simulink model "ScriptDemo"  (R2022b)
settings: configuration reference "TmVcThermal_Configuration_sub" (kept outside this file)
undefined symbols (not defined in the file): aaaa, bbbb, cTmComprCtrl_D_u8HvacFlowTable_db, cTmComprCtrl_D_u8HvacFlowTable_sw, cTmComprCtrl_n_i16ChillCmpIMax, cTmComprCtrl_n_i16ChillCmpIMin, cTmComprCtrl_n_i16ChillCmpIMin666, cTmComprCtrl_n_i16ChillCmpPMax, cTmComprCtrl_n_i16ChillCmpPMin, cTmComprCtrl_n_i16CmpChillCoolRpmKiMax, cTmComprCtrl_n_i16CmpChillCoolRpmKiMin, cTmComprCtrl_n_i16CmpChillCoolRpmKpMax, cTmComprCtrl_n_i16CmpChillCoolRpmKpMin, cTmComprCtrl_n_i16CmpCoolRpmKiMax, cTmComprCtrl_n_i16CmpCoolRpmKiMin, cTmComprCtrl_n_i16CmpCoolRpmKpMax, cTmComprCtrl_n_i16CmpCoolRpmKpMin, cTmComprCtrl_n_i16SM4CmpHeatKiMax, cTmComprCtrl_n_i16SM4CmpHeatKiMin, cTmComprCtrl_n_i16SM4CmpHeatKpMax, cTmComprCtrl_n_i16SM4CmpHeatKpMin, cTmComprCtrl_n_i16SM5CmpHeatKiMax, cTmComprCtrl_n_i16SM5CmpHeatKiMin, cTmComprCtrl_n_i16SM5CmpHeatKpMax, cTmComprCtrl_n_i16SM5CmpHeatKpMin, cTmComprCtrl_n_i16SM6CmpHeatKiMax, cTmComprCtrl_n_i16SM6CmpHeatKiMin, cTmComprCtrl_n_i16SM6CmpHeatKpMax, cTmComprCtrl_n_i16SM6CmpHeatKpMin, cTmComprCtrl_n_u16CmpMaxSpdFanFltLimt, cTmComprCtrl_n_u16CmpMaxSpdLoSidePFltLimt, cTmComprCtrl_n_u16CmpMaxSpdSensorFltLimt, cTmComprCtrl_n_u16CompMinRpm, cTmComprCtrl_n_u16CompRpmIncThres, cTmComprCtrl_t_u16BattCooltFFPeriod, cTmComprCtrl_t_u16BattCooltPIPeriod, cTmComprCtrl_t_u16CmpCoolFFPeriod, cTmComprCtrl_t_u16CmpCoolPIPeriod, cTmComprCtrl_t_u16CoolCmpChillFFPeriod, cTmComprCtrl_t_u16CoolCmpChillPIPeriod, cTmComprCtrl_t_u16SM4CmpHeatFFPeriod, cTmComprCtrl_t_u16SM4CmpHeatPIPeriod, cTmComprCtrl_t_u16SM5CmpHeatFFPeriod, cTmComprCtrl_t_u16SM5CmpHeatPIPeriod, cTmComprCtrl_t_u16SM6CmpHeatFFPeriod, cTmComprCtrl_t_u16SM6CmpHeatPIPeriod, cTmComprCtrl_Te_EvapClearInteg, cTmComprCtrl_Te_i16HpReqTempSaturoffset, cTmComprCtrl_Te_i16SatLpReplaceDiff, cTmComprCtrl_Te_i16SM3BatDiffStartEvapDecOffset, cTmComprCtrl_Te_i16SM3EvapLo, cTmComprCtrl_Te_i16SM3TBatDiffEntEvapDecOffset, cTmComprCtrl_Te_i16SM3TBatDiffEntEvapDecOffsetQuit, cTmComprCtrl_Te_s32ErrCmpChillPIContinueCoolH, cTmComprCtrl_Te_s32ErrCmpChillPIContinueCoolL, cTmComprCtrl_Te_s32ErrCmpPIContinueChillH, cTmComprCtrl_Te_s32ErrCmpPIContinueChillL, cTmComprCtrl_Te_s32ErrCmpPIContinueCoolH, cTmComprCtrl_Te_s32ErrCmpPIContinueCoolL, cTmComprCtrl_Te_s32ErrCmpPIContinueHeatH ... (+398)
libraries: simulink x782, PCMULib x640, simulink_need_slupdate x4
(part 16 of 41)

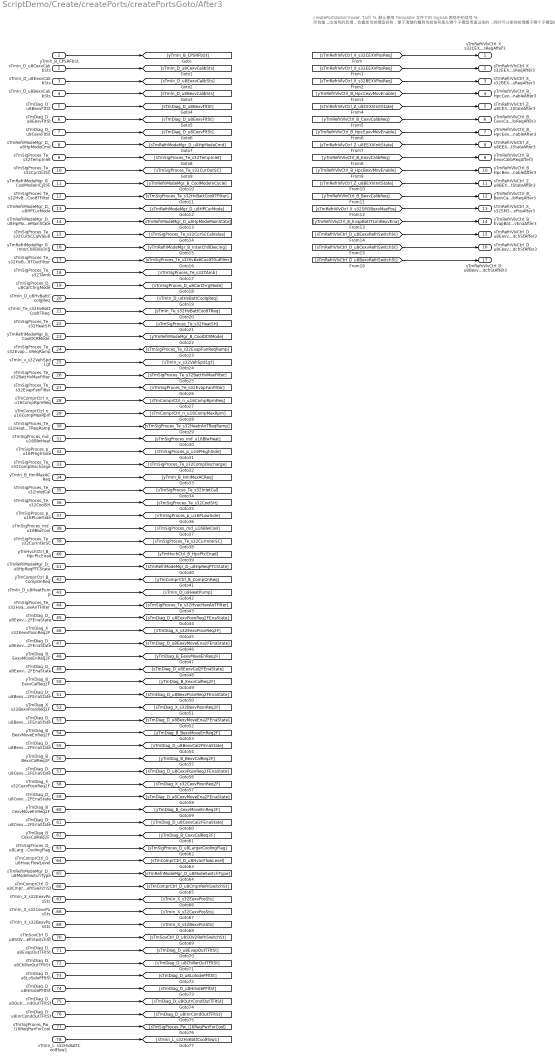
== system ScriptDemo/Create/createPorts/createPortsGoto/After3 ==
  note: createPortsGoto('mode','tail')
      | % 默认使用 Template 文件下的 Signals 表格中的信号
      | % 所有输出信号的后缀，会叠加当前模型名称，便于清楚的看到当前信号是从哪个子模型传递过来的，同时可以保持前缀属于哪个子模型的
  yTmIn_B_CPSRFbSt : Inport  OutDataTypeStr=boolean
  sTmIn_D_u8CexvCalibSts : Inport  Port=2  OutDataTypeStr=uint8
  sTmIn_D_u8EexvCalibSts : Inport  Port=3  OutDataTypeStr=uint8
  sTmIn_D_u8BexvCalibSts : Inport  Port=4  OutDataTypeStr=uint8
  sTmDiag_D_u8BexvFltSt : Inport  Port=5  OutDataTypeStr=uint8
  sTmDiag_D_u8EexvFltSt : Inport  Port=6  OutDataTypeStr=uint8
  sTmDiag_D_u8CexvFltSt : Inport  Port=7  OutDataTypeStr=uint8
  sTmRefriModeMgr_D_u8HpModeCmd : Inport  Port=8  OutDataTypeStr=uint8
  sTmSigProces_Te_s32TempInlet : Inport  Port=9  OutDataTypeStr=single
  sTmSigProces_Te_s32CurOutSC : Inport  Port=10  OutDataTypeStr=single
  yTmRefriModeMgr_B_CoolModeInCycle : Inport  Port=11  OutDataTypeStr=boolean
  sTmSigProces_Te_s32HvBattCooltTFilter : Inport  Port=12  OutDataTypeStr=single
  sTmRefriModeMgr_D_u8HPCurMode : Inport  Port=13  OutDataTypeStr=uint8
  sTmRefriModeMgr_D_u8HpModeMainState : Inport  Port=14  OutDataTypeStr=uint8
  sTmSigProces_Te_s32CurSCCalValue : Inport  Port=15  OutDataTypeStr=single
  yTmRefriModeMgr_B_InterChillDeicing : Inport  Port=16  OutDataTypeStr=boolean
  sTmSigProces_Te_s32HvBattCooltTOutFilter : Inport  Port=17  OutDataTypeStr=single
  sTmSigProces_Te_s32TAmb : Inport  Port=18  OutDataTypeStr=single
  sTmSigProces_D_u8CarChrgMode : Inport  Port=19  OutDataTypeStr=uint8
  sTmIn_D_u8HvBattCoolgReq : Inport  Port=20  OutDataTypeStr=uint8
  sTmIn_Te_s32HvBattCooltTReq : Inport  Port=21  OutDataTypeStr=single
  sTmSigProces_Te_s32HeatSH : Inport  Port=22  OutDataTypeStr=single
  yTmRefriModeMgr_B_CoolOCRMode : Inport  Port=23  OutDataTypeStr=boolean
  sTmSigProces_Te_s32EvapFanReqRamp : Inport  Port=24  OutDataTypeStr=single
  sTmIn_v_s32VehSpdLgt : Inport  Port=25  OutDataTypeStr=single
  sTmSigProces_Te_s32BattHvMaxFilter : Inport  Port=26  OutDataTypeStr=single
  sTmSigProces_Te_s32EvapFanFilter : Inport  Port=27  OutDataTypeStr=single
  sTmComprCtrl_n_u16CompRpmReq : Inport  Port=28  OutDataTypeStr=uint16
  sTmComprCtrl_n_u16CompMaxRpm : Inport  Port=29  OutDataTypeStr=uint16
  sTmSigProces_Te_s32HeatrAirTReqRamp : Inport  Port=30  OutDataTypeStr=single
  sTmSigProces_md_u16BlwHeat : Inport  Port=31  OutDataTypeStr=uint16
  sTmSigProces_p_u16PHighSide : Inport  Port=32  OutDataTypeStr=uint16
  sTmSigProces_Te_s32CompDischarge : Inport  Port=33  OutDataTypeStr=single
  yTmIn_B_HmiMaxACReq : Inport  Port=34  OutDataTypeStr=boolean
  sTmSigProces_Te_s32InletCal : Inport  Port=35  OutDataTypeStr=single
  sTmSigProces_Te_s32CoolSH : Inport  Port=36  OutDataTypeStr=single
  sTmSigProces_p_u16PLowSide : Inport  Port=37  OutDataTypeStr=uint16
  sTmSigProces_md_u16BlwCool : Inport  Port=38  OutDataTypeStr=uint16
  sTmSigProces_Te_s32CurInterSC : Inport  Port=39  OutDataTypeStr=single
  yTmHvchCtrl_B_HpcPtcEnad : Inport  Port=40  OutDataTypeStr=boolean
  sTmRefriModeMgr_D_u8HpReqPTCState : Inport  Port=41  OutDataTypeStr=uint8
  yTmComprCtrl_B_CompOnReq : Inport  Port=42  OutDataTypeStr=boolean
  sTmIn_D_u8HeatPump : Inport  Port=43  OutDataTypeStr=uint8
  sTmSigProces_Te_s32HvacHexAirTFilter : Inport  Port=44  OutDataTypeStr=single
  sTmDiag_D_u8EexvPosnReq2FEnaState : Inport  Port=45  OutDataTypeStr=uint8
  sTmDiag_X_s32EexvPosnReq2F : Inport  Port=46  OutDataTypeStr=single
  sTmDiag_D_u8EexvMoveEna2FEnaState : Inport  Port=47  OutDataTypeStr=uint8
  yTmDiag_B_EexvMoveEnReq2F : Inport  Port=48  OutDataTypeStr=boolean
  sTmDiag_D_u8EexvCal2FEnaState : Inport  Port=49  OutDataTypeStr=uint8
  yTmDiag_B_EexvCalReq2F : Inport  Port=50  OutDataTypeStr=boolean
  sTmDiag_D_u8BexvPosnReq2FEnaState : Inport  Port=51  OutDataTypeStr=uint8
  sTmDiag_X_s32BexvPosnReq2F : Inport  Port=52  OutDataTypeStr=single
  sTmDiag_D_u8BexvMoveEna2FEnaState : Inport  Port=53  OutDataTypeStr=uint8
  yTmDiag_B_BexvMoveEnReq2F : Inport  Port=54  OutDataTypeStr=boolean
  sTmDiag_D_u8BexvCal2FEnaState : Inport  Port=55  OutDataTypeStr=uint8
  yTmDiag_B_BexvCalReq2F : Inport  Port=56  OutDataTypeStr=boolean
  sTmDiag_D_u8CexvPosnReq2FEnaState : Inport  Port=57  OutDataTypeStr=uint8
  sTmDiag_X_s32CexvPosnReq2F : Inport  Port=58  OutDataTypeStr=single
  sTmDiag_D_u8CexvMoveEna2FEnaState : Inport  Port=59  OutDataTypeStr=uint8
  yTmDiag_B_CexvMoveEnReq2F : Inport  Port=60  OutDataTypeStr=boolean
  sTmDiag_D_u8CexvCal2FEnaState : Inport  Port=61  OutDataTypeStr=uint8
  yTmDiag_B_CexvCalReq2F : Inport  Port=62  OutDataTypeStr=boolean
  sTmSigProces_D_u8LargerCoolingFlag : Inport  Port=63  OutDataTypeStr=uint8
  sTmComprCtrl_D_u8HvacFlowLevel : Inport  Port=64  OutDataTypeStr=uint8
  sTmRefriModeMgr_D_u8ModeSwitchType : Inport  Port=65  OutDataTypeStr=uint8
  sTmComprCtrl_D_u8CmprRefriSwitchSt : Inport  Port=66  OutDataTypeStr=uint8
  sTmIn_X_s32EexvPosSts : Inport  Port=67  OutDataTypeStr=single
  sTmIn_X_s32CexvPosSts : Inport  Port=68  OutDataTypeStr=single
  sTmIn_X_s32BexvPosSts : Inport  Port=69  OutDataTypeStr=single
  sTmSovCtrl_D_u8SOV2RefriSwitchSt : Inport  Port=70  OutDataTypeStr=uint8
  sTmDiag_D_u8EvapOutTFltSt : Inport  Port=71  OutDataTypeStr=uint8
  sTmDiag_D_u8ChillerOutTFltSt : Inport  Port=72  OutDataTypeStr=uint8
  sTmDiag_D_u8LoSidePFltSt : Inport  Port=73  OutDataTypeStr=uint8
  sTmDiag_D_u8HiSidePFltSt : Inport  Port=74  OutDataTypeStr=uint8
  sTmDiag_D_u8OutrCondOutTFltSt : Inport  Port=75  OutDataTypeStr=uint8
  sTmDiag_D_u8InrCondOutTFltSt : Inport  Port=76  OutDataTypeStr=uint8
  sTmSigProces_Pw_i16ReqPwrForCool : Inport  Port=77  OutDataTypeStr=int16
  sTmIn_L_s32HvBattCoolFlow1 : Inport  Port=78  OutDataTypeStr=single
  sTmRefriVlvCtrl_X_s32CEXVPosReqAfter3 : Outport  OutDataTypeStr=single
  sTmRefriVlvCtrl_X_s32EEXVPosReqAfter3 : Outport  Port=2  OutDataTypeStr=single
  sTmRefriVlvCtrl_X_s32BEXVPosReqAfter3 : Outport  Port=3  OutDataTypeStr=single
  yTmRefriVlvCtrl_B_HpcCexvMovEnableAfter3 : Outport  Port=4  OutDataTypeStr=boolean
  sTmRefriVlvCtrl_Z_u8CEXVInitStateAfter3 : Outport  Port=5  OutDataTypeStr=uint8
  yTmRefriVlvCtrl_B_CexvCalibReqAfter3 : Outport  Port=6  OutDataTypeStr=boolean
  yTmRefriVlvCtrl_B_HpcEexvMovEnableAfter3 : Outport  Port=7  OutDataTypeStr=boolean
  sTmRefriVlvCtrl_Z_u8EEXVInitStateAfter3 : Outport  Port=8  OutDataTypeStr=uint8
  yTmRefriVlvCtrl_B_EexvCalibReqAfter3 : Outport  Port=9  OutDataTypeStr=boolean
  yTmRefriVlvCtrl_B_HpcBexvMovEnableAfter3 : Outport  Port=10  OutDataTypeStr=boolean
  sTmRefriVlvCtrl_Z_u8BEXVInitStateAfter3 : Outport  Port=11  OutDataTypeStr=uint8
  yTmRefriVlvCtrl_B_BexvCalibReqAfter3 : Outport  Port=12  OutDataTypeStr=boolean
  sTmRefriVlvCtrl_X_s32SM3BexvMaxPosAfter3 : Outport  Port=13  OutDataTypeStr=single
  yTmRefriVlvCtrl_B_EvapBattTLimBexvEnaAfter3 : Outport  Port=14  OutDataTypeStr=boolean
  sTmRefriVlvCtrl_D_u8EexvRefriSwitchStAfter3 : Outport  Port=15  OutDataTypeStr=uint8
  sTmRefriVlvCtrl_D_u8CexvRefriSwitchStAfter3 : Outport  Port=16  OutDataTypeStr=uint8
  sTmRefriVlvCtrl_D_u8BexvRefriSwitchStAfter3 : Outport  Port=17  OutDataTypeStr=uint8
  wires:
  yTmIn_B_CPSRFbSt/1 -> [yTmIn_B_CPSRFbSt]
  sTmIn_D_u8CexvCalibSts/1 -> [sTmIn_D_u8CexvCalibSts]
  sTmIn_D_u8EexvCalibSts/1 -> [sTmIn_D_u8EexvCalibSts]
  sTmIn_D_u8BexvCalibSts/1 -> [sTmIn_D_u8BexvCalibSts]
  sTmDiag_D_u8BexvFltSt/1 -> [sTmDiag_D_u8BexvFltSt]
  sTmDiag_D_u8EexvFltSt/1 -> [sTmDiag_D_u8EexvFltSt]
  sTmDiag_D_u8CexvFltSt/1 -> [sTmDiag_D_u8CexvFltSt]
  sTmRefriModeMgr_D_u8HpModeCmd/1 -> [sTmRefriModeMgr_D_u8HpModeCmd]
  sTmSigProces_Te_s32TempInlet/1 -> [sTmSigProces_Te_s32TempInlet]
  sTmSigProces_Te_s32CurOutSC/1 -> [sTmSigProces_Te_s32CurOutSC]
  yTmRefriModeMgr_B_CoolModeInCycle/1 -> [yTmRefriModeMgr_B_CoolModeInCycle]
  sTmSigProces_Te_s32HvBattCooltTFilter/1 -> [sTmSigProces_Te_s32HvBattCooltTFilter]
  sTmRefriModeMgr_D_u8HPCurMode/1 -> [sTmRefriModeMgr_D_u8HPCurMode]
  sTmRefriModeMgr_D_u8HpModeMainState/1 -> [sTmRefriModeMgr_D_u8HpModeMainState]
  sTmSigProces_Te_s32CurSCCalValue/1 -> [sTmSigProces_Te_s32CurSCCalValue]
  yTmRefriModeMgr_B_InterChillDeicing/1 -> [yTmRefriModeMgr_B_InterChillDeicing]
  sTmSigProces_Te_s32HvBattCooltTOutFilter/1 -> [sTmSigProces_Te_s32HvBattCooltTOutFilter]
  sTmSigProces_Te_s32TAmb/1 -> [sTmSigProces_Te_s32TAmb]
  sTmSigProces_D_u8CarChrgMode/1 -> [sTmSigProces_D_u8CarChrgMode]
  sTmIn_D_u8HvBattCoolgReq/1 -> [sTmIn_D_u8HvBattCoolgReq]
  sTmIn_Te_s32HvBattCooltTReq/1 -> [sTmIn_Te_s32HvBattCooltTReq]
  sTmSigProces_Te_s32HeatSH/1 -> [sTmSigProces_Te_s32HeatSH]
  yTmRefriModeMgr_B_CoolOCRMode/1 -> [yTmRefriModeMgr_B_CoolOCRMode]
  sTmSigProces_Te_s32EvapFanReqRamp/1 -> [sTmSigProces_Te_s32EvapFanReqRamp]
  sTmIn_v_s32VehSpdLgt/1 -> [sTmIn_v_s32VehSpdLgt]
  sTmSigProces_Te_s32BattHvMaxFilter/1 -> [sTmSigProces_Te_s32BattHvMaxFilter]
  sTmSigProces_Te_s32EvapFanFilter/1 -> [sTmSigProces_Te_s32EvapFanFilter]
  sTmComprCtrl_n_u16CompRpmReq/1 -> [sTmComprCtrl_n_u16CompRpmReq]
  sTmComprCtrl_n_u16CompMaxRpm/1 -> [sTmComprCtrl_n_u16CompMaxRpm]
  sTmSigProces_Te_s32HeatrAirTReqRamp/1 -> [sTmSigProces_Te_s32HeatrAirTReqRamp]
  sTmSigProces_md_u16BlwHeat/1 -> [sTmSigProces_md_u16BlwHeat]
  sTmSigProces_p_u16PHighSide/1 -> [sTmSigProces_p_u16PHighSide]
  sTmSigProces_Te_s32CompDischarge/1 -> [sTmSigProces_Te_s32CompDischarge]
  yTmIn_B_HmiMaxACReq/1 -> [yTmIn_B_HmiMaxACReq]
  sTmSigProces_Te_s32InletCal/1 -> [sTmSigProces_Te_s32InletCal]
  sTmSigProces_Te_s32CoolSH/1 -> [sTmSigProces_Te_s32CoolSH]
  sTmSigProces_p_u16PLowSide/1 -> [sTmSigProces_p_u16PLowSide]
  sTmSigProces_md_u16BlwCool/1 -> [sTmSigProces_md_u16BlwCool]
  sTmSigProces_Te_s32CurInterSC/1 -> [sTmSigProces_Te_s32CurInterSC]
  yTmHvchCtrl_B_HpcPtcEnad/1 -> [yTmHvchCtrl_B_HpcPtcEnad]
  sTmRefriModeMgr_D_u8HpReqPTCState/1 -> [sTmRefriModeMgr_D_u8HpReqPTCState]
  yTmComprCtrl_B_CompOnReq/1 -> [yTmComprCtrl_B_CompOnReq]
  sTmIn_D_u8HeatPump/1 -> [sTmIn_D_u8HeatPump]
  sTmSigProces_Te_s32HvacHexAirTFilter/1 -> [sTmSigProces_Te_s32HvacHexAirTFilter]
  sTmDiag_D_u8EexvPosnReq2FEnaState/1 -> [sTmDiag_D_u8EexvPosnReq2FEnaState]
  sTmDiag_X_s32EexvPosnReq2F/1 -> [sTmDiag_X_s32EexvPosnReq2F]
  sTmDiag_D_u8EexvMoveEna2FEnaState/1 -> [sTmDiag_D_u8EexvMoveEna2FEnaState]
  yTmDiag_B_EexvMoveEnReq2F/1 -> [yTmDiag_B_EexvMoveEnReq2F]
  sTmDiag_D_u8EexvCal2FEnaState/1 -> [sTmDiag_D_u8EexvCal2FEnaState]
  yTmDiag_B_EexvCalReq2F/1 -> [yTmDiag_B_EexvCalReq2F]
  sTmDiag_D_u8BexvPosnReq2FEnaState/1 -> [sTmDiag_D_u8BexvPosnReq2FEnaState]
  sTmDiag_X_s32BexvPosnReq2F/1 -> [sTmDiag_X_s32BexvPosnReq2F]
  sTmDiag_D_u8BexvMoveEna2FEnaState/1 -> [sTmDiag_D_u8BexvMoveEna2FEnaState]
  yTmDiag_B_BexvMoveEnReq2F/1 -> [yTmDiag_B_BexvMoveEnReq2F]
  sTmDiag_D_u8BexvCal2FEnaState/1 -> [sTmDiag_D_u8BexvCal2FEnaState]
  yTmDiag_B_BexvCalReq2F/1 -> [yTmDiag_B_BexvCalReq2F]
  sTmDiag_D_u8CexvPosnReq2FEnaState/1 -> [sTmDiag_D_u8CexvPosnReq2FEnaState]
  sTmDiag_X_s32CexvPosnReq2F/1 -> [sTmDiag_X_s32CexvPosnReq2F]
  sTmDiag_D_u8CexvMoveEna2FEnaState/1 -> [sTmDiag_D_u8CexvMoveEna2FEnaState]
  yTmDiag_B_CexvMoveEnReq2F/1 -> [yTmDiag_B_CexvMoveEnReq2F]
  sTmDiag_D_u8CexvCal2FEnaState/1 -> [sTmDiag_D_u8CexvCal2FEnaState]
  yTmDiag_B_CexvCalReq2F/1 -> [yTmDiag_B_CexvCalReq2F]
  sTmSigProces_D_u8LargerCoolingFlag/1 -> [sTmSigProces_D_u8LargerCoolingFlag]
  sTmComprCtrl_D_u8HvacFlowLevel/1 -> [sTmComprCtrl_D_u8HvacFlowLevel]
  sTmRefriModeMgr_D_u8ModeSwitchType/1 -> [sTmRefriModeMgr_D_u8ModeSwitchType]
  sTmComprCtrl_D_u8CmprRefriSwitchSt/1 -> [sTmComprCtrl_D_u8CmprRefriSwitchSt]
  sTmIn_X_s32EexvPosSts/1 -> [sTmIn_X_s32EexvPosSts]
  sTmIn_X_s32CexvPosSts/1 -> [sTmIn_X_s32CexvPosSts]
  sTmIn_X_s32BexvPosSts/1 -> [sTmIn_X_s32BexvPosSts]
  sTmSovCtrl_D_u8SOV2RefriSwitchSt/1 -> [sTmSovCtrl_D_u8SOV2RefriSwitchSt]
  sTmDiag_D_u8EvapOutTFltSt/1 -> [sTmDiag_D_u8EvapOutTFltSt]
  sTmDiag_D_u8ChillerOutTFltSt/1 -> [sTmDiag_D_u8ChillerOutTFltSt]
  sTmDiag_D_u8LoSidePFltSt/1 -> [sTmDiag_D_u8LoSidePFltSt]
  sTmDiag_D_u8HiSidePFltSt/1 -> [sTmDiag_D_u8HiSidePFltSt]
  sTmDiag_D_u8OutrCondOutTFltSt/1 -> [sTmDiag_D_u8OutrCondOutTFltSt]
  sTmDiag_D_u8InrCondOutTFltSt/1 -> [sTmDiag_D_u8InrCondOutTFltSt]
  sTmSigProces_Pw_i16ReqPwrForCool/1 -> [sTmSigProces_Pw_i16ReqPwrForCool]
  sTmIn_L_s32HvBattCoolFlow1/1 -> [sTmIn_L_s32HvBattCoolFlow1]
  [sTmRefriVlvCtrl_X_s32CEXVPosReq] -> sTmRefriVlvCtrl_X_s32CEXVPosReqAfter3/1
  [sTmRefriVlvCtrl_X_s32EEXVPosReq] -> sTmRefriVlvCtrl_X_s32EEXVPosReqAfter3/1
  [sTmRefriVlvCtrl_X_s32BEXVPosReq] -> sTmRefriVlvCtrl_X_s32BEXVPosReqAfter3/1
  [yTmRefriVlvCtrl_B_HpcCexvMovEnable] -> yTmRefriVlvCtrl_B_HpcCexvMovEnableAfter3/1
  [sTmRefriVlvCtrl_Z_u8CEXVInitState] -> sTmRefriVlvCtrl_Z_u8CEXVInitStateAfter3/1
  [yTmRefriVlvCtrl_B_CexvCalibReq] -> yTmRefriVlvCtrl_B_CexvCalibReqAfter3/1
  [yTmRefriVlvCtrl_B_HpcEexvMovEnable] -> yTmRefriVlvCtrl_B_HpcEexvMovEnableAfter3/1
  [sTmRefriVlvCtrl_Z_u8EEXVInitState] -> sTmRefriVlvCtrl_Z_u8EEXVInitStateAfter3/1
  [yTmRefriVlvCtrl_B_EexvCalibReq] -> yTmRefriVlvCtrl_B_EexvCalibReqAfter3/1
  [yTmRefriVlvCtrl_B_HpcBexvMovEnable] -> yTmRefriVlvCtrl_B_HpcBexvMovEnableAfter3/1
  [sTmRefriVlvCtrl_Z_u8BEXVInitState] -> sTmRefriVlvCtrl_Z_u8BEXVInitStateAfter3/1
  [yTmRefriVlvCtrl_B_BexvCalibReq] -> yTmRefriVlvCtrl_B_BexvCalibReqAfter3/1
  [sTmRefriVlvCtrl_X_s32SM3BexvMaxPos] -> sTmRefriVlvCtrl_X_s32SM3BexvMaxPosAfter3/1
  [yTmRefriVlvCtrl_B_EvapBattTLimBexvEna] -> yTmRefriVlvCtrl_B_EvapBattTLimBexvEnaAfter3/1
  [sTmRefriVlvCtrl_D_u8EexvRefriSwitchSt] -> sTmRefriVlvCtrl_D_u8EexvRefriSwitchStAfter3/1
  [sTmRefriVlvCtrl_D_u8CexvRefriSwitchSt] -> sTmRefriVlvCtrl_D_u8CexvRefriSwitchStAfter3/1
  [sTmRefriVlvCtrl_D_u8BexvRefriSwitchSt] -> sTmRefriVlvCtrl_D_u8BexvRefriSwitchStAfter3/1

== system ScriptDemo/Create/createPorts/createPortsGotoUpdate/After ==
  note: createPortsGotoUpdate()
      |
      | % 在此路径下执行
      | % 保持原有的信号名
  sTmIn_Pw_s32HvCoolgAllwd : Inport  OutDataTypeStr=single
  xTmComprCtrl_B_CompOnReqCompOn : Inport  Port=2  OutDataTypeStr=boolean
  AllowedPower : Subsystem
  sTmComprCtrl_Pw_s32ElacCmprMaxState : Outport  OutDataTypeStr=single
  yTmComprCtrl_B_HpcCoolgLimd : Outport  Port=2  OutDataTypeStr=boolean
  wires:
  [xTmComprCtrl_B_CompOnReqCompOn] -> AllowedPower/2(xTmComprCtrl_B_CompOnReqCompOn)
  [sTmIn_Pw_s32HvCoolgAllwd] -> AllowedPower/1(sTmIn_Pw_s32HvCoolgAllwd)
  AllowedPower/2(yTmComprCtrl_B_HpcCoolgLimd) -> [yTmComprCtrl_B_HpcCoolgLimd]
  AllowedPower/1(sTmComprCtrl_Pw_s32ElacCmprMaxState) -> [sTmComprCtrl_Pw_s32ElacCmprMaxState]
  sTmIn_Pw_s32HvCoolgAllwd/1 -> [sTmIn_Pw_s32HvCoolgAllwd]
  xTmComprCtrl_B_CompOnReqCompOn/1 -> [xTmComprCtrl_B_CompOnReqCompOn]
  [sTmComprCtrl_Pw_s32ElacCmprMaxState] -> sTmComprCtrl_Pw_s32ElacCmprMaxState/1
  [yTmComprCtrl_B_HpcCoolgLimd] -> yTmComprCtrl_B_HpcCoolgLimd/1

== system ScriptDemo/Create/createPorts/createPortsGotoUpdate/After1 ==
  note: createPortsGotoUpdate( 'mode' , 'pre' )
      |
      | % 在此路径下执行
      | % 使用当前子模型名称作为前缀
  sTmIn_Pw_s32HvCoolgAllwd : Inport  OutDataTypeStr=single
  xTmComprCtrl_B_CompOnReqCompOn : Inport  Port=2  OutDataTypeStr=boolean
  AllowedPower : Subsystem
  rAfter1_Pw_s32ElacCmprMaxState : Outport  OutDataTypeStr=single
  xAfter1_B_HpcCoolgLimd : Outport  Port=2  OutDataTypeStr=boolean
  wires:
  AllowedPower/1(sTmComprCtrl_Pw_s32ElacCmprMaxState) -> [sTmComprCtrl_Pw_s32ElacCmprMaxState]
  [xTmComprCtrl_B_CompOnReqCompOn] -> AllowedPower/2(xTmComprCtrl_B_CompOnReqCompOn)
  [sTmIn_Pw_s32HvCoolgAllwd] -> AllowedPower/1(sTmIn_Pw_s32HvCoolgAllwd)
  AllowedPower/2(yTmComprCtrl_B_HpcCoolgLimd) -> [yTmComprCtrl_B_HpcCoolgLimd]
  sTmIn_Pw_s32HvCoolgAllwd/1 -> [sTmIn_Pw_s32HvCoolgAllwd]
  xTmComprCtrl_B_CompOnReqCompOn/1 -> [xTmComprCtrl_B_CompOnReqCompOn]
  [sTmComprCtrl_Pw_s32ElacCmprMaxState] -> rAfter1_Pw_s32ElacCmprMaxState/1
  [yTmComprCtrl_B_HpcCoolgLimd] -> xAfter1_B_HpcCoolgLimd/1

== system ScriptDemo/Create/createPorts/createPortsGotoUpdate/Before ==
  AllowedPower : Subsystem
  wires:
  [xTmComprCtrl_B_CompOnReqCompOn] -> AllowedPower/2(xTmComprCtrl_B_CompOnReqCompOn)
  [sTmIn_Pw_s32HvCoolgAllwd] -> AllowedPower/1(sTmIn_Pw_s32HvCoolgAllwd)
  AllowedPower/2(yTmComprCtrl_B_HpcCoolgLimd) -> [yTmComprCtrl_B_HpcCoolgLimd]
  AllowedPower/1(sTmComprCtrl_Pw_s32ElacCmprMaxState) -> [sTmComprCtrl_Pw_s32ElacCmprMaxState]

== system ScriptDemo/Create/createPorts/createPortsGotoUpdateLoop/After ==
  sTmIn_Pw_s32HvCoolgAllwd : Inport  OutDataTypeStr=single  OutputFunctionCall=on
  xTmComprCtrl_B_CompOnReqCompOn : Inport  Port=2  OutDataTypeStr=boolean
  xTmComprCtrl_B_AddedSignal : Inport  Port=3  OutDataTypeStr=boolean
  Level3 : Subsystem
  sTmComprCtrl_Pw_s32ElacCmprMaxState : Outport  OutDataTypeStr=single
  yTmComprCtrl_B_HpcCoolgLimd : Outport  Port=2  OutDataTypeStr=boolean
  wires:
  sTmIn_Pw_s32HvCoolgAllwd/1 -> Level3/1(sTmIn_Pw_s32HvCoolgAllwd)  "sTmIn_Pw_s32HvCoolgAllwd"
  xTmComprCtrl_B_CompOnReqCompOn/1 -> Level3/2(xTmComprCtrl_B_CompOnReqCompOn)  "xTmComprCtrl_B_CompOnReqCompOn"
  Level3/1(sTmComprCtrl_Pw_s32ElacCmprMaxState) -> sTmComprCtrl_Pw_s32ElacCmprMaxState/1  "sTmComprCtrl_Pw_s32ElacCmprMaxState"
  Level3/2(yTmComprCtrl_B_HpcCoolgLimd) -> yTmComprCtrl_B_HpcCoolgLimd/1  "yTmComprCtrl_B_HpcCoolgLimd"
  xTmComprCtrl_B_AddedSignal/1 -> Level3/3(xTmComprCtrl_B_AddedSignal)  "xTmComprCtrl_B_AddedSignal"

== system ScriptDemo/Create/createPorts/createPortsGotoUpdateLoop/Before ==
  sTmIn_Pw_s32HvCoolgAllwd : Inport  OutDataTypeStr=single  OutputFunctionCall=on
  xTmComprCtrl_B_CompOnReqCompOn : Inport  Port=2  OutDataTypeStr=boolean
  Level3 : Subsystem
  sTmComprCtrl_Pw_s32ElacCmprMaxState : Outport  OutDataTypeStr=single
  yTmComprCtrl_B_HpcCoolgLimd : Outport  Port=2  OutDataTypeStr=boolean
  wires:
  sTmIn_Pw_s32HvCoolgAllwd/1 -> Level3/1(sTmIn_Pw_s32HvCoolgAllwd)  "sTmIn_Pw_s32HvCoolgAllwd"
  xTmComprCtrl_B_CompOnReqCompOn/1 -> Level3/2(xTmComprCtrl_B_CompOnReqCompOn)  "xTmComprCtrl_B_CompOnReqCompOn"
  Level3/1(sTmComprCtrl_Pw_s32ElacCmprMaxState) -> sTmComprCtrl_Pw_s32ElacCmprMaxState/1  "sTmComprCtrl_Pw_s32ElacCmprMaxState"
  Level3/2(yTmComprCtrl_B_HpcCoolgLimd) -> yTmComprCtrl_B_HpcCoolgLimd/1  "yTmComprCtrl_B_HpcCoolgLimd"

== system ScriptDemo/Create/createSigOnLine/After/Before ==
  note: % 目的: 为输出端口创建debug 及对应的输入模块
      | [cnt] = createDebug(gcs)
  sTmRefriVlvCtrl_X_s32CEXVPosReqIn : Inport  OutDataTypeStr=single
  sTmRefriVlvCtrl_X_s32EEXVPosReqIn : Inport  Port=2  OutDataTypeStr=single
  sTmRefriVlvCtrl_X_s32BEXVPosReqIn : Inport  Port=3  OutDataTypeStr=single
  yTmRefriVlvCtrl_B_HpcCexvMovEnableIn : Inport  Port=4  OutDataTypeStr=boolean
  sTmRefriVlvCtrl_Z_u8CEXVInitStateIn : Inport  Port=5  OutDataTypeStr=uint8
  yTmRefriVlvCtrl_B_CexvCalibReqIn : Inport  Port=6  OutDataTypeStr=boolean
  yTmRefriVlvCtrl_B_HpcEexvMovEnableIn : Inport  Port=7  OutDataTypeStr=boolean
  sTmRefriVlvCtrl_Z_u8EEXVInitStateIn : Inport  Port=8  OutDataTypeStr=uint8
  yTmRefriVlvCtrl_B_EexvCalibReqIn : Inport  Port=9  OutDataTypeStr=boolean
  yTmRefriVlvCtrl_B_HpcBexvMovEnableIn : Inport  Port=10  OutDataTypeStr=boolean
  sTmRefriVlvCtrl_Z_u8BEXVInitStateIn : Inport  Port=11  OutDataTypeStr=uint8
  yTmRefriVlvCtrl_B_BexvCalibReqIn : Inport  Port=12  OutDataTypeStr=boolean
  sTmRefriVlvCtrl_X_s32SM3BexvMaxPosIn : Inport  Port=13  OutDataTypeStr=single
  yTmRefriVlvCtrl_B_EvapBattTLimBexvEnaIn : Inport  Port=14  OutDataTypeStr=boolean
  sTmRefriVlvCtrl_D_u8EexvRefriSwitchStIn : Inport  Port=15  OutDataTypeStr=uint8
  sTmRefriVlvCtrl_D_u8CexvRefriSwitchStIn : Inport  Port=16  OutDataTypeStr=uint8
  sTmRefriVlvCtrl_D_u8BexvRefriSwitchStIn : Inport  Port=17  OutDataTypeStr=uint8
  OutDebug : PCMULib/Interface/OutdebugRvs  SWI=cTmRefriVlvCtrl_X_s32CEXVPosReq_sw  DBI=cTmRefriVlvCtrl_X_s32CEXVPosReq_db
      settings: SourceProductName=PCMULib
  OutDebug1 : PCMULib/Interface/OutdebugRvs  SWI=cTmRefriVlvCtrl_X_s32EEXVPosReq_sw  DBI=cTmRefriVlvCtrl_X_s32EEXVPosReq_db
      settings: SourceProductName=PCMULib
  OutDebug10 : PCMULib/Interface/OutdebugRvs  SWI=cTmRefriVlvCtrl_Z_u8BEXVInitState_sw  DBI=cTmRefriVlvCtrl_Z_u8BEXVInitState_db
      settings: SourceProductName=PCMULib
  OutDebug11 : PCMULib/Interface/OutdebugRvs  SWI=cTmRefriVlvCtrl_B_BexvCalibReq_sw  DBI=cTmRefriVlvCtrl_B_BexvCalibReq_db
      settings: SourceProductName=PCMULib
  OutDebug12 : PCMULib/Interface/OutdebugRvs  SWI=cTmRefriVlvCtrl_X_s32SM3BexvMaxPos_sw  DBI=cTmRefriVlvCtrl_X_s32SM3BexvMaxPos_db
      settings: SourceProductName=PCMULib
  OutDebug13 : PCMULib/Interface/OutdebugRvs  SWI=cTmRefriVlvCtrl_B_EvapBattTLimBexvEna_sw  DBI=cTmRefriVlvCtrl_B_EvapBattTLimBexvEna_db
      settings: SourceProductName=PCMULib
  OutDebug14 : PCMULib/Interface/OutdebugRvs  SWI=cTmRefriVlvCtrl_D_u8EexvRefriSwitchSt_sw  DBI=cTmRefriVlvCtrl_D_u8EexvRefriSwitchSt_db
      settings: SourceProductName=PCMULib
  OutDebug15 : PCMULib/Interface/OutdebugRvs  SWI=cTmRefriVlvCtrl_D_u8CexvRefriSwitchSt_sw  DBI=cTmRefriVlvCtrl_D_u8CexvRefriSwitchSt_db
      settings: SourceProductName=PCMULib
  OutDebug16 : PCMULib/Interface/OutdebugRvs  SWI=cTmRefriVlvCtrl_D_u8BexvRefriSwitchSt_sw  DBI=cTmRefriVlvCtrl_D_u8BexvRefriSwitchSt_db
      settings: SourceProductName=PCMULib
  OutDebug2 : PCMULib/Interface/OutdebugRvs  SWI=cTmRefriVlvCtrl_X_s32BEXVPosReq_sw  DBI=cTmRefriVlvCtrl_X_s32BEXVPosReq_db
      settings: SourceProductName=PCMULib
  OutDebug3 : PCMULib/Interface/OutdebugRvs  SWI=cTmRefriVlvCtrl_B_HpcCexvMovEnable_sw  DBI=cTmRefriVlvCtrl_B_HpcCexvMovEnable_db
      settings: SourceProductName=PCMULib
  OutDebug4 : PCMULib/Interface/OutdebugRvs  SWI=cTmRefriVlvCtrl_Z_u8CEXVInitState_sw  DBI=cTmRefriVlvCtrl_Z_u8CEXVInitState_db
      settings: SourceProductName=PCMULib
  OutDebug5 : PCMULib/Interface/OutdebugRvs  SWI=cTmRefriVlvCtrl_B_CexvCalibReq_sw  DBI=cTmRefriVlvCtrl_B_CexvCalibReq_db
      settings: SourceProductName=PCMULib
  OutDebug6 : PCMULib/Interface/OutdebugRvs  SWI=cTmRefriVlvCtrl_B_HpcEexvMovEnable_sw  DBI=cTmRefriVlvCtrl_B_HpcEexvMovEnable_db
      settings: SourceProductName=PCMULib
  OutDebug7 : PCMULib/Interface/OutdebugRvs  SWI=cTmRefriVlvCtrl_Z_u8EEXVInitState_sw  DBI=cTmRefriVlvCtrl_Z_u8EEXVInitState_db
      settings: SourceProductName=PCMULib
  OutDebug8 : PCMULib/Interface/OutdebugRvs  SWI=cTmRefriVlvCtrl_B_EexvCalibReq_sw  DBI=cTmRefriVlvCtrl_B_EexvCalibReq_db
      settings: SourceProductName=PCMULib
  OutDebug9 : PCMULib/Interface/OutdebugRvs  SWI=cTmRefriVlvCtrl_B_HpcBexvMovEnable_sw  DBI=cTmRefriVlvCtrl_B_HpcBexvMovEnable_db
      settings: SourceProductName=PCMULib
  sTmRefriVlvCtrl_X_s32CEXVPosReq : Outport  OutDataTypeStr=single
  sTmRefriVlvCtrl_X_s32EEXVPosReq : Outport  Port=2  OutDataTypeStr=single
  sTmRefriVlvCtrl_X_s32BEXVPosReq : Outport  Port=3  OutDataTypeStr=single
  yTmRefriVlvCtrl_B_HpcCexvMovEnable : Outport  Port=4  OutDataTypeStr=boolean
  sTmRefriVlvCtrl_Z_u8CEXVInitState : Outport  Port=5  OutDataTypeStr=uint8
  yTmRefriVlvCtrl_B_CexvCalibReq : Outport  Port=6  OutDataTypeStr=boolean
  yTmRefriVlvCtrl_B_HpcEexvMovEnable : Outport  Port=7  OutDataTypeStr=boolean
  sTmRefriVlvCtrl_Z_u8EEXVInitState : Outport  Port=8  OutDataTypeStr=uint8
  yTmRefriVlvCtrl_B_EexvCalibReq : Outport  Port=9  OutDataTypeStr=boolean
  yTmRefriVlvCtrl_B_HpcBexvMovEnable : Outport  Port=10  OutDataTypeStr=boolean
  sTmRefriVlvCtrl_Z_u8BEXVInitState : Outport  Port=11  OutDataTypeStr=uint8
  yTmRefriVlvCtrl_B_BexvCalibReq : Outport  Port=12  OutDataTypeStr=boolean
  sTmRefriVlvCtrl_X_s32SM3BexvMaxPos : Outport  Port=13  OutDataTypeStr=single
  yTmRefriVlvCtrl_B_EvapBattTLimBexvEna : Outport  Port=14  OutDataTypeStr=boolean
  sTmRefriVlvCtrl_D_u8EexvRefriSwitchSt : Outport  Port=15  OutDataTypeStr=uint8
  sTmRefriVlvCtrl_D_u8CexvRefriSwitchSt : Outport  Port=16  OutDataTypeStr=uint8
  sTmRefriVlvCtrl_D_u8BexvRefriSwitchSt : Outport  Port=17  OutDataTypeStr=uint8
  wires:
  sTmRefriVlvCtrl_X_s32SM3BexvMaxPosIn/1 -> OutDebug12/1
  OutDebug12/1 -> sTmRefriVlvCtrl_X_s32SM3BexvMaxPos/1
  sTmRefriVlvCtrl_X_s32BEXVPosReqIn/1 -> OutDebug2/1
  OutDebug2/1 -> sTmRefriVlvCtrl_X_s32BEXVPosReq/1
  OutDebug16/1 -> sTmRefriVlvCtrl_D_u8BexvRefriSwitchSt/1
  sTmRefriVlvCtrl_D_u8EexvRefriSwitchStIn/1 -> OutDebug14/1
  OutDebug5/1 -> yTmRefriVlvCtrl_B_CexvCalibReq/1
  OutDebug3/1 -> yTmRefriVlvCtrl_B_HpcCexvMovEnable/1
  sTmRefriVlvCtrl_Z_u8CEXVInitStateIn/1 -> OutDebug4/1
  OutDebug4/1 -> sTmRefriVlvCtrl_Z_u8CEXVInitState/1
  sTmRefriVlvCtrl_D_u8BexvRefriSwitchStIn/1 -> OutDebug16/1
  OutDebug1/1 -> sTmRefriVlvCtrl_X_s32EEXVPosReq/1
  OutDebug14/1 -> sTmRefriVlvCtrl_D_u8EexvRefriSwitchSt/1
  yTmRefriVlvCtrl_B_CexvCalibReqIn/1 -> OutDebug5/1
  sTmRefriVlvCtrl_X_s32EEXVPosReqIn/1 -> OutDebug1/1
  yTmRefriVlvCtrl_B_HpcCexvMovEnableIn/1 -> OutDebug3/1
  yTmRefriVlvCtrl_B_EvapBattTLimBexvEnaIn/1 -> OutDebug13/1
  OutDebug13/1 -> yTmRefriVlvCtrl_B_EvapBattTLimBexvEna/1
  sTmRefriVlvCtrl_Z_u8BEXVInitStateIn/1 -> OutDebug10/1
  OutDebug10/1 -> sTmRefriVlvCtrl_Z_u8BEXVInitState/1
  sTmRefriVlvCtrl_D_u8CexvRefriSwitchStIn/1 -> OutDebug15/1
  OutDebug15/1 -> sTmRefriVlvCtrl_D_u8CexvRefriSwitchSt/1
  OutDebug/1 -> sTmRefriVlvCtrl_X_s32CEXVPosReq/1
  OutDebug7/1 -> sTmRefriVlvCtrl_Z_u8EEXVInitState/1
  OutDebug8/1 -> yTmRefriVlvCtrl_B_EexvCalibReq/1
  yTmRefriVlvCtrl_B_EexvCalibReqIn/1 -> OutDebug8/1
  sTmRefriVlvCtrl_X_s32CEXVPosReqIn/1 -> OutDebug/1
  OutDebug6/1 -> yTmRefriVlvCtrl_B_HpcEexvMovEnable/1
  yTmRefriVlvCtrl_B_HpcEexvMovEnableIn/1 -> OutDebug6/1
  sTmRefriVlvCtrl_Z_u8EEXVInitStateIn/1 -> OutDebug7/1
  yTmRefriVlvCtrl_B_HpcBexvMovEnableIn/1 -> OutDebug9/1
  OutDebug9/1 -> yTmRefriVlvCtrl_B_HpcBexvMovEnable/1
  yTmRefriVlvCtrl_B_BexvCalibReqIn/1 -> OutDebug11/1
  OutDebug11/1 -> yTmRefriVlvCtrl_B_BexvCalibReq/1

== system ScriptDemo/Create/createSigOnLine/After2/Before ==
  note: % 目的: 为输出端口创建debug 及对应的输入模块
      | [cnt] = createDebug(gcs)
  sTmRefriVlvCtrl_X_s32CEXVPosReqIn : Inport  OutDataTypeStr=single
  sTmRefriVlvCtrl_X_s32EEXVPosReqIn : Inport  Port=2  OutDataTypeStr=single
  sTmRefriVlvCtrl_X_s32BEXVPosReqIn : Inport  Port=3  OutDataTypeStr=single
  yTmRefriVlvCtrl_B_HpcCexvMovEnableIn : Inport  Port=4  OutDataTypeStr=boolean
  sTmRefriVlvCtrl_Z_u8CEXVInitStateIn : Inport  Port=5  OutDataTypeStr=uint8
  yTmRefriVlvCtrl_B_CexvCalibReqIn : Inport  Port=6  OutDataTypeStr=boolean
  yTmRefriVlvCtrl_B_HpcEexvMovEnableIn : Inport  Port=7  OutDataTypeStr=boolean
  sTmRefriVlvCtrl_Z_u8EEXVInitStateIn : Inport  Port=8  OutDataTypeStr=uint8
  yTmRefriVlvCtrl_B_EexvCalibReqIn : Inport  Port=9  OutDataTypeStr=boolean
  yTmRefriVlvCtrl_B_HpcBexvMovEnableIn : Inport  Port=10  OutDataTypeStr=boolean
  sTmRefriVlvCtrl_Z_u8BEXVInitStateIn : Inport  Port=11  OutDataTypeStr=uint8
  yTmRefriVlvCtrl_B_BexvCalibReqIn : Inport  Port=12  OutDataTypeStr=boolean
  sTmRefriVlvCtrl_X_s32SM3BexvMaxPosIn : Inport  Port=13  OutDataTypeStr=single
  yTmRefriVlvCtrl_B_EvapBattTLimBexvEnaIn : Inport  Port=14  OutDataTypeStr=boolean
  sTmRefriVlvCtrl_D_u8EexvRefriSwitchStIn : Inport  Port=15  OutDataTypeStr=uint8
  sTmRefriVlvCtrl_D_u8CexvRefriSwitchStIn : Inport  Port=16  OutDataTypeStr=uint8
  sTmRefriVlvCtrl_D_u8BexvRefriSwitchStIn : Inport  Port=17  OutDataTypeStr=uint8
  OutDebug : PCMULib/Interface/OutdebugRvs  SWI=cTmRefriVlvCtrl_X_s32CEXVPosReq_sw  DBI=cTmRefriVlvCtrl_X_s32CEXVPosReq_db
      settings: SourceProductName=PCMULib
  OutDebug1 : PCMULib/Interface/OutdebugRvs  SWI=cTmRefriVlvCtrl_X_s32EEXVPosReq_sw  DBI=cTmRefriVlvCtrl_X_s32EEXVPosReq_db
      settings: SourceProductName=PCMULib
  OutDebug10 : PCMULib/Interface/OutdebugRvs  SWI=cTmRefriVlvCtrl_Z_u8BEXVInitState_sw  DBI=cTmRefriVlvCtrl_Z_u8BEXVInitState_db
      settings: SourceProductName=PCMULib
  OutDebug11 : PCMULib/Interface/OutdebugRvs  SWI=cTmRefriVlvCtrl_B_BexvCalibReq_sw  DBI=cTmRefriVlvCtrl_B_BexvCalibReq_db
      settings: SourceProductName=PCMULib
  OutDebug12 : PCMULib/Interface/OutdebugRvs  SWI=cTmRefriVlvCtrl_X_s32SM3BexvMaxPos_sw  DBI=cTmRefriVlvCtrl_X_s32SM3BexvMaxPos_db
      settings: SourceProductName=PCMULib
  OutDebug13 : PCMULib/Interface/OutdebugRvs  SWI=cTmRefriVlvCtrl_B_EvapBattTLimBexvEna_sw  DBI=cTmRefriVlvCtrl_B_EvapBattTLimBexvEna_db
      settings: SourceProductName=PCMULib
  OutDebug14 : PCMULib/Interface/OutdebugRvs  SWI=cTmRefriVlvCtrl_D_u8EexvRefriSwitchSt_sw  DBI=cTmRefriVlvCtrl_D_u8EexvRefriSwitchSt_db
      settings: SourceProductName=PCMULib
  OutDebug15 : PCMULib/Interface/OutdebugRvs  SWI=cTmRefriVlvCtrl_D_u8CexvRefriSwitchSt_sw  DBI=cTmRefriVlvCtrl_D_u8CexvRefriSwitchSt_db
      settings: SourceProductName=PCMULib
  OutDebug16 : PCMULib/Interface/OutdebugRvs  SWI=cTmRefriVlvCtrl_D_u8BexvRefriSwitchSt_sw  DBI=cTmRefriVlvCtrl_D_u8BexvRefriSwitchSt_db
      settings: SourceProductName=PCMULib
  OutDebug2 : PCMULib/Interface/OutdebugRvs  SWI=cTmRefriVlvCtrl_X_s32BEXVPosReq_sw  DBI=cTmRefriVlvCtrl_X_s32BEXVPosReq_db
      settings: SourceProductName=PCMULib
  OutDebug3 : PCMULib/Interface/OutdebugRvs  SWI=cTmRefriVlvCtrl_B_HpcCexvMovEnable_sw  DBI=cTmRefriVlvCtrl_B_HpcCexvMovEnable_db
      settings: SourceProductName=PCMULib
  OutDebug4 : PCMULib/Interface/OutdebugRvs  SWI=cTmRefriVlvCtrl_Z_u8CEXVInitState_sw  DBI=cTmRefriVlvCtrl_Z_u8CEXVInitState_db
      settings: SourceProductName=PCMULib
  OutDebug5 : PCMULib/Interface/OutdebugRvs  SWI=cTmRefriVlvCtrl_B_CexvCalibReq_sw  DBI=cTmRefriVlvCtrl_B_CexvCalibReq_db
      settings: SourceProductName=PCMULib
  OutDebug6 : PCMULib/Interface/OutdebugRvs  SWI=cTmRefriVlvCtrl_B_HpcEexvMovEnable_sw  DBI=cTmRefriVlvCtrl_B_HpcEexvMovEnable_db
      settings: SourceProductName=PCMULib
  OutDebug7 : PCMULib/Interface/OutdebugRvs  SWI=cTmRefriVlvCtrl_Z_u8EEXVInitState_sw  DBI=cTmRefriVlvCtrl_Z_u8EEXVInitState_db
      settings: SourceProductName=PCMULib
  OutDebug8 : PCMULib/Interface/OutdebugRvs  SWI=cTmRefriVlvCtrl_B_EexvCalibReq_sw  DBI=cTmRefriVlvCtrl_B_EexvCalibReq_db
      settings: SourceProductName=PCMULib
  OutDebug9 : PCMULib/Interface/OutdebugRvs  SWI=cTmRefriVlvCtrl_B_HpcBexvMovEnable_sw  DBI=cTmRefriVlvCtrl_B_HpcBexvMovEnable_db
      settings: SourceProductName=PCMULib
  sTmRefriVlvCtrl_X_s32CEXVPosReq : Outport  OutDataTypeStr=single
  sTmRefriVlvCtrl_X_s32EEXVPosReq : Outport  Port=2  OutDataTypeStr=single
  sTmRefriVlvCtrl_X_s32BEXVPosReq : Outport  Port=3  OutDataTypeStr=single
  yTmRefriVlvCtrl_B_HpcCexvMovEnable : Outport  Port=4  OutDataTypeStr=boolean
  sTmRefriVlvCtrl_Z_u8CEXVInitState : Outport  Port=5  OutDataTypeStr=uint8
  yTmRefriVlvCtrl_B_CexvCalibReq : Outport  Port=6  OutDataTypeStr=boolean
  yTmRefriVlvCtrl_B_HpcEexvMovEnable : Outport  Port=7  OutDataTypeStr=boolean
  sTmRefriVlvCtrl_Z_u8EEXVInitState : Outport  Port=8  OutDataTypeStr=uint8
  yTmRefriVlvCtrl_B_EexvCalibReq : Outport  Port=9  OutDataTypeStr=boolean
  yTmRefriVlvCtrl_B_HpcBexvMovEnable : Outport  Port=10  OutDataTypeStr=boolean
  sTmRefriVlvCtrl_Z_u8BEXVInitState : Outport  Port=11  OutDataTypeStr=uint8
  yTmRefriVlvCtrl_B_BexvCalibReq : Outport  Port=12  OutDataTypeStr=boolean
  sTmRefriVlvCtrl_X_s32SM3BexvMaxPos : Outport  Port=13  OutDataTypeStr=single
  yTmRefriVlvCtrl_B_EvapBattTLimBexvEna : Outport  Port=14  OutDataTypeStr=boolean
  sTmRefriVlvCtrl_D_u8EexvRefriSwitchSt : Outport  Port=15  OutDataTypeStr=uint8
  sTmRefriVlvCtrl_D_u8CexvRefriSwitchSt : Outport  Port=16  OutDataTypeStr=uint8
  sTmRefriVlvCtrl_D_u8BexvRefriSwitchSt : Outport  Port=17  OutDataTypeStr=uint8
  wires:
  sTmRefriVlvCtrl_X_s32SM3BexvMaxPosIn/1 -> OutDebug12/1
  OutDebug12/1 -> sTmRefriVlvCtrl_X_s32SM3BexvMaxPos/1
  sTmRefriVlvCtrl_X_s32BEXVPosReqIn/1 -> OutDebug2/1
  OutDebug2/1 -> sTmRefriVlvCtrl_X_s32BEXVPosReq/1
  OutDebug16/1 -> sTmRefriVlvCtrl_D_u8BexvRefriSwitchSt/1
  sTmRefriVlvCtrl_D_u8EexvRefriSwitchStIn/1 -> OutDebug14/1
  OutDebug5/1 -> yTmRefriVlvCtrl_B_CexvCalibReq/1
  OutDebug3/1 -> yTmRefriVlvCtrl_B_HpcCexvMovEnable/1
  sTmRefriVlvCtrl_Z_u8CEXVInitStateIn/1 -> OutDebug4/1
  OutDebug4/1 -> sTmRefriVlvCtrl_Z_u8CEXVInitState/1
  sTmRefriVlvCtrl_D_u8BexvRefriSwitchStIn/1 -> OutDebug16/1
  OutDebug1/1 -> sTmRefriVlvCtrl_X_s32EEXVPosReq/1
  OutDebug14/1 -> sTmRefriVlvCtrl_D_u8EexvRefriSwitchSt/1
  yTmRefriVlvCtrl_B_CexvCalibReqIn/1 -> OutDebug5/1
  sTmRefriVlvCtrl_X_s32EEXVPosReqIn/1 -> OutDebug1/1
  yTmRefriVlvCtrl_B_HpcCexvMovEnableIn/1 -> OutDebug3/1
  yTmRefriVlvCtrl_B_EvapBattTLimBexvEnaIn/1 -> OutDebug13/1
  OutDebug13/1 -> yTmRefriVlvCtrl_B_EvapBattTLimBexvEna/1
  sTmRefriVlvCtrl_Z_u8BEXVInitStateIn/1 -> OutDebug10/1
  OutDebug10/1 -> sTmRefriVlvCtrl_Z_u8BEXVInitState/1
  sTmRefriVlvCtrl_D_u8CexvRefriSwitchStIn/1 -> OutDebug15/1
  OutDebug15/1 -> sTmRefriVlvCtrl_D_u8CexvRefriSwitchSt/1
  OutDebug/1 -> sTmRefriVlvCtrl_X_s32CEXVPosReq/1
  OutDebug7/1 -> sTmRefriVlvCtrl_Z_u8EEXVInitState/1
  OutDebug8/1 -> yTmRefriVlvCtrl_B_EexvCalibReq/1
  yTmRefriVlvCtrl_B_EexvCalibReqIn/1 -> OutDebug8/1
  sTmRefriVlvCtrl_X_s32CEXVPosReqIn/1 -> OutDebug/1
  OutDebug6/1 -> yTmRefriVlvCtrl_B_HpcEexvMovEnable/1
  yTmRefriVlvCtrl_B_HpcEexvMovEnableIn/1 -> OutDebug6/1
  sTmRefriVlvCtrl_Z_u8EEXVInitStateIn/1 -> OutDebug7/1
  yTmRefriVlvCtrl_B_HpcBexvMovEnableIn/1 -> OutDebug9/1
  OutDebug9/1 -> yTmRefriVlvCtrl_B_HpcBexvMovEnable/1
  yTmRefriVlvCtrl_B_BexvCalibReqIn/1 -> OutDebug11/1
  OutDebug11/1 -> yTmRefriVlvCtrl_B_BexvCalibReq/1

== system ScriptDemo/Create/createSigOnLine/After3/Before ==
  note: % 目的: 为输出端口创建debug 及对应的输入模块
      | [cnt] = createDebug(gcs)
  sTmRefriVlvCtrl_X_s32CEXVPosReqIn : Inport  OutDataTypeStr=single
  sTmRefriVlvCtrl_X_s32EEXVPosReqIn : Inport  Port=2  OutDataTypeStr=single
  sTmRefriVlvCtrl_X_s32BEXVPosReqIn : Inport  Port=3  OutDataTypeStr=single
  yTmRefriVlvCtrl_B_HpcCexvMovEnableIn : Inport  Port=4  OutDataTypeStr=boolean
  sTmRefriVlvCtrl_Z_u8CEXVInitStateIn : Inport  Port=5  OutDataTypeStr=uint8
  yTmRefriVlvCtrl_B_CexvCalibReqIn : Inport  Port=6  OutDataTypeStr=boolean
  yTmRefriVlvCtrl_B_HpcEexvMovEnableIn : Inport  Port=7  OutDataTypeStr=boolean
  sTmRefriVlvCtrl_Z_u8EEXVInitStateIn : Inport  Port=8  OutDataTypeStr=uint8
  yTmRefriVlvCtrl_B_EexvCalibReqIn : Inport  Port=9  OutDataTypeStr=boolean
  yTmRefriVlvCtrl_B_HpcBexvMovEnableIn : Inport  Port=10  OutDataTypeStr=boolean
  sTmRefriVlvCtrl_Z_u8BEXVInitStateIn : Inport  Port=11  OutDataTypeStr=uint8
  yTmRefriVlvCtrl_B_BexvCalibReqIn : Inport  Port=12  OutDataTypeStr=boolean
  sTmRefriVlvCtrl_X_s32SM3BexvMaxPosIn : Inport  Port=13  OutDataTypeStr=single
  yTmRefriVlvCtrl_B_EvapBattTLimBexvEnaIn : Inport  Port=14  OutDataTypeStr=boolean
  sTmRefriVlvCtrl_D_u8EexvRefriSwitchStIn : Inport  Port=15  OutDataTypeStr=uint8
  sTmRefriVlvCtrl_D_u8CexvRefriSwitchStIn : Inport  Port=16  OutDataTypeStr=uint8
  sTmRefriVlvCtrl_D_u8BexvRefriSwitchStIn : Inport  Port=17  OutDataTypeStr=uint8
  OutDebug : PCMULib/Interface/OutdebugRvs  SWI=cTmRefriVlvCtrl_X_s32CEXVPosReq_sw  DBI=cTmRefriVlvCtrl_X_s32CEXVPosReq_db
      settings: SourceProductName=PCMULib
  OutDebug1 : PCMULib/Interface/OutdebugRvs  SWI=cTmRefriVlvCtrl_X_s32EEXVPosReq_sw  DBI=cTmRefriVlvCtrl_X_s32EEXVPosReq_db
      settings: SourceProductName=PCMULib
  OutDebug10 : PCMULib/Interface/OutdebugRvs  SWI=cTmRefriVlvCtrl_Z_u8BEXVInitState_sw  DBI=cTmRefriVlvCtrl_Z_u8BEXVInitState_db
      settings: SourceProductName=PCMULib
  OutDebug11 : PCMULib/Interface/OutdebugRvs  SWI=cTmRefriVlvCtrl_B_BexvCalibReq_sw  DBI=cTmRefriVlvCtrl_B_BexvCalibReq_db
      settings: SourceProductName=PCMULib
  OutDebug12 : PCMULib/Interface/OutdebugRvs  SWI=cTmRefriVlvCtrl_X_s32SM3BexvMaxPos_sw  DBI=cTmRefriVlvCtrl_X_s32SM3BexvMaxPos_db
      settings: SourceProductName=PCMULib
  OutDebug13 : PCMULib/Interface/OutdebugRvs  SWI=cTmRefriVlvCtrl_B_EvapBattTLimBexvEna_sw  DBI=cTmRefriVlvCtrl_B_EvapBattTLimBexvEna_db
      settings: SourceProductName=PCMULib
  OutDebug14 : PCMULib/Interface/OutdebugRvs  SWI=cTmRefriVlvCtrl_D_u8EexvRefriSwitchSt_sw  DBI=cTmRefriVlvCtrl_D_u8EexvRefriSwitchSt_db
      settings: SourceProductName=PCMULib
  OutDebug15 : PCMULib/Interface/OutdebugRvs  SWI=cTmRefriVlvCtrl_D_u8CexvRefriSwitchSt_sw  DBI=cTmRefriVlvCtrl_D_u8CexvRefriSwitchSt_db
      settings: SourceProductName=PCMULib
  OutDebug16 : PCMULib/Interface/OutdebugRvs  SWI=cTmRefriVlvCtrl_D_u8BexvRefriSwitchSt_sw  DBI=cTmRefriVlvCtrl_D_u8BexvRefriSwitchSt_db
      settings: SourceProductName=PCMULib
  OutDebug2 : PCMULib/Interface/OutdebugRvs  SWI=cTmRefriVlvCtrl_X_s32BEXVPosReq_sw  DBI=cTmRefriVlvCtrl_X_s32BEXVPosReq_db
      settings: SourceProductName=PCMULib
  OutDebug3 : PCMULib/Interface/OutdebugRvs  SWI=cTmRefriVlvCtrl_B_HpcCexvMovEnable_sw  DBI=cTmRefriVlvCtrl_B_HpcCexvMovEnable_db
      settings: SourceProductName=PCMULib
  OutDebug4 : PCMULib/Interface/OutdebugRvs  SWI=cTmRefriVlvCtrl_Z_u8CEXVInitState_sw  DBI=cTmRefriVlvCtrl_Z_u8CEXVInitState_db
      settings: SourceProductName=PCMULib
  OutDebug5 : PCMULib/Interface/OutdebugRvs  SWI=cTmRefriVlvCtrl_B_CexvCalibReq_sw  DBI=cTmRefriVlvCtrl_B_CexvCalibReq_db
      settings: SourceProductName=PCMULib
  OutDebug6 : PCMULib/Interface/OutdebugRvs  SWI=cTmRefriVlvCtrl_B_HpcEexvMovEnable_sw  DBI=cTmRefriVlvCtrl_B_HpcEexvMovEnable_db
      settings: SourceProductName=PCMULib
  OutDebug7 : PCMULib/Interface/OutdebugRvs  SWI=cTmRefriVlvCtrl_Z_u8EEXVInitState_sw  DBI=cTmRefriVlvCtrl_Z_u8EEXVInitState_db
      settings: SourceProductName=PCMULib
  OutDebug8 : PCMULib/Interface/OutdebugRvs  SWI=cTmRefriVlvCtrl_B_EexvCalibReq_sw  DBI=cTmRefriVlvCtrl_B_EexvCalibReq_db
      settings: SourceProductName=PCMULib
  OutDebug9 : PCMULib/Interface/OutdebugRvs  SWI=cTmRefriVlvCtrl_B_HpcBexvMovEnable_sw  DBI=cTmRefriVlvCtrl_B_HpcBexvMovEnable_db
      settings: SourceProductName=PCMULib
  sTmRefriVlvCtrl_X_s32CEXVPosReq : Outport  OutDataTypeStr=single
  sTmRefriVlvCtrl_X_s32EEXVPosReq : Outport  Port=2  OutDataTypeStr=single
  sTmRefriVlvCtrl_X_s32BEXVPosReq : Outport  Port=3  OutDataTypeStr=single
  yTmRefriVlvCtrl_B_HpcCexvMovEnable : Outport  Port=4  OutDataTypeStr=boolean
  sTmRefriVlvCtrl_Z_u8CEXVInitState : Outport  Port=5  OutDataTypeStr=uint8
  yTmRefriVlvCtrl_B_CexvCalibReq : Outport  Port=6  OutDataTypeStr=boolean
  yTmRefriVlvCtrl_B_HpcEexvMovEnable : Outport  Port=7  OutDataTypeStr=boolean
  sTmRefriVlvCtrl_Z_u8EEXVInitState : Outport  Port=8  OutDataTypeStr=uint8
  yTmRefriVlvCtrl_B_EexvCalibReq : Outport  Port=9  OutDataTypeStr=boolean
  yTmRefriVlvCtrl_B_HpcBexvMovEnable : Outport  Port=10  OutDataTypeStr=boolean
  sTmRefriVlvCtrl_Z_u8BEXVInitState : Outport  Port=11  OutDataTypeStr=uint8
  yTmRefriVlvCtrl_B_BexvCalibReq : Outport  Port=12  OutDataTypeStr=boolean
  sTmRefriVlvCtrl_X_s32SM3BexvMaxPos : Outport  Port=13  OutDataTypeStr=single
  yTmRefriVlvCtrl_B_EvapBattTLimBexvEna : Outport  Port=14  OutDataTypeStr=boolean
  sTmRefriVlvCtrl_D_u8EexvRefriSwitchSt : Outport  Port=15  OutDataTypeStr=uint8
  sTmRefriVlvCtrl_D_u8CexvRefriSwitchSt : Outport  Port=16  OutDataTypeStr=uint8
  sTmRefriVlvCtrl_D_u8BexvRefriSwitchSt : Outport  Port=17  OutDataTypeStr=uint8
  wires:
  sTmRefriVlvCtrl_X_s32SM3BexvMaxPosIn/1 -> OutDebug12/1
  OutDebug12/1 -> sTmRefriVlvCtrl_X_s32SM3BexvMaxPos/1
  sTmRefriVlvCtrl_X_s32BEXVPosReqIn/1 -> OutDebug2/1
  OutDebug2/1 -> sTmRefriVlvCtrl_X_s32BEXVPosReq/1
  OutDebug16/1 -> sTmRefriVlvCtrl_D_u8BexvRefriSwitchSt/1
  sTmRefriVlvCtrl_D_u8EexvRefriSwitchStIn/1 -> OutDebug14/1
  OutDebug5/1 -> yTmRefriVlvCtrl_B_CexvCalibReq/1
  OutDebug3/1 -> yTmRefriVlvCtrl_B_HpcCexvMovEnable/1
  sTmRefriVlvCtrl_Z_u8CEXVInitStateIn/1 -> OutDebug4/1
  OutDebug4/1 -> sTmRefriVlvCtrl_Z_u8CEXVInitState/1
  sTmRefriVlvCtrl_D_u8BexvRefriSwitchStIn/1 -> OutDebug16/1
  OutDebug1/1 -> sTmRefriVlvCtrl_X_s32EEXVPosReq/1
  OutDebug14/1 -> sTmRefriVlvCtrl_D_u8EexvRefriSwitchSt/1
  yTmRefriVlvCtrl_B_CexvCalibReqIn/1 -> OutDebug5/1
  sTmRefriVlvCtrl_X_s32EEXVPosReqIn/1 -> OutDebug1/1
  yTmRefriVlvCtrl_B_HpcCexvMovEnableIn/1 -> OutDebug3/1
  yTmRefriVlvCtrl_B_EvapBattTLimBexvEnaIn/1 -> OutDebug13/1
  OutDebug13/1 -> yTmRefriVlvCtrl_B_EvapBattTLimBexvEna/1
  sTmRefriVlvCtrl_Z_u8BEXVInitStateIn/1 -> OutDebug10/1
  OutDebug10/1 -> sTmRefriVlvCtrl_Z_u8BEXVInitState/1
  sTmRefriVlvCtrl_D_u8CexvRefriSwitchStIn/1 -> OutDebug15/1
  OutDebug15/1 -> sTmRefriVlvCtrl_D_u8CexvRefriSwitchSt/1
  OutDebug/1 -> sTmRefriVlvCtrl_X_s32CEXVPosReq/1
  OutDebug7/1 -> sTmRefriVlvCtrl_Z_u8EEXVInitState/1
  OutDebug8/1 -> yTmRefriVlvCtrl_B_EexvCalibReq/1
  yTmRefriVlvCtrl_B_EexvCalibReqIn/1 -> OutDebug8/1
  sTmRefriVlvCtrl_X_s32CEXVPosReqIn/1 -> OutDebug/1
  OutDebug6/1 -> yTmRefriVlvCtrl_B_HpcEexvMovEnable/1
  yTmRefriVlvCtrl_B_HpcEexvMovEnableIn/1 -> OutDebug6/1
  sTmRefriVlvCtrl_Z_u8EEXVInitStateIn/1 -> OutDebug7/1
  yTmRefriVlvCtrl_B_HpcBexvMovEnableIn/1 -> OutDebug9/1
  OutDebug9/1 -> yTmRefriVlvCtrl_B_HpcBexvMovEnable/1
  yTmRefriVlvCtrl_B_BexvCalibReqIn/1 -> OutDebug11/1
  OutDebug11/1 -> yTmRefriVlvCtrl_B_BexvCalibReq/1
